simulink library "powerlib_models"  (Simulink 6.0)
settings: Solver=ode45  SolverMode=SingleTasking  StartTime=0.0  StopTime=10.0  RelTol=1e-3
values from neighbouring files (symbols this model uses):
  Ts = get(handles.edit1,'string')    [powergui.m]
undefined symbols (not defined in the file or in its folder): A, a0, a1, a2, a3, a4, a5, Ac, Amplitude, Amplitudes, B, BaseCurrent, BaseFlux, Bc, C, Capacitance, Cc, Columns, ConnectionType, Cs, ctrl, current, Current, damp, Dc, Dd, DiscIntNeverNeededParam, dref, dwo, exc, excAxis, F, Flux, fnom, Frequency, FreqVps, Gain1, gate, GH, GHd, GI, GId, GL, GLd, H, HarmonicGeneration, HT, hyd, I1_init, ib, ib2, Id1o, Inductance, InitialFlux, InitialSlope, io, Iq1o, isfinite, j, J ... (+138)
libraries: powerlib_models x32, powerlib_extras x4
(part 4 of 11)

== system powerlib_models/Discrete/PSS ==
  note: Power System Stabilizer (PSS)
      | (Discrete generic model)
  In : Inport  Port=1  LatchInput=off
  Lead-Lag #1 : Subsystem  AncestorBlock=|  mask(Discrete Lead-Lag Controller){T1=T1n, T2=T1d, V_Init=0, Ts=Ts}
      | powerlib_extras/Discrete 
      | Control Blocks/Discrete
      | Lead-Lag
      mask prompts: T1 "Time constant T1 (s):"; T2 "Time constant T2 (s):"; V_Init "Initial input and output:"; Ts "Sample time (s):"
      mask help:
      | This block implements a discrete lead-lag controller:
      |
      |          1+T1s
      | H(s)= ------
      |          1+T2s
      |
      | States are initialized according to initial input anf output value so that simulation starts in steady state.
      mask init: same as powerlib_models/Discrete/Excitation_System/Lead Lag Compensator tc.s+1 / tb.s+1
      mask Display: disp('1+T1s\n---\n1+T2s')
  Lead-Lag #2 : Subsystem  AncestorBlock=|  mask(Discrete Lead-Lag Controller){T1=T2n, T2=T2d, V_Init=0, Ts=Ts}
      | powerlib_extras/Discrete 
      | Control Blocks/Discrete
      | Lead-Lag
      mask prompts: T1 "Time constant T1 (s):"; T2 "Time constant T2 (s):"; V_Init "Initial input and output:"; Ts "Sample time (s):"
      mask help:
      | This block implements a discrete lead-lag controller:
      |
      |          1+T1s
      | H(s)= ------
      |          1+T2s
      |
      | States are initialized according to initial input anf output value so that simulation starts in steady state.
      mask init: same as powerlib_models/Discrete/Excitation_System/Lead Lag Compensator tc.s+1 / tb.s+1
      mask Display: disp('1+T1s\n---\n1+T2s')
  "Limiter " : Saturate  UpperLimit=VSlimits(2)  LowerLimit=VSlimits(1)
  Overall Gain : Gain  Gain=K  SaturateOnIntegerOverflow=on
  "Sensor " : Subsystem  AncestorBlock=|  mask(Discrete 1st-Order Filter){FilterType=Lowpass, Tc=Tsensor, Ts=Ts, Initialize=on, Vac_Init=[0 0 60], Vdc_Init=Vinit, PlotResponse=off, param1=[1 500 0.1]}
      | powerlib_extras/Discrete 
      | Control Blocks/Discrete
      | 1st-Order
      | Discrete Filter
      mask prompts: FilterType "Filter Type:"; Tc "Time constant (s):"; Ts "Sample time:"; Initialize "Initialize filter states"; Vac_Init "AC initial input: [ Mag  Phase(degrees)  Freq(Hz) ]"; Vdc_Init "DC Initial input:"; PlotResponse "Plot filter response"; param1 "Frequency range(Hz) : [Start  End  Inc.]"
      mask init:
      | switch FilterType
      | case 1, % Lowpass
      |        X=[0 1 2 3 4];
      |        Y=[-2 -2 -3 -4 -4];
      |        numc=1;
      |        denc=[Tc 1];
      |  case 2,   % Highpass
      |        X=[0 1 2 3 4];
      |        Y=[-4 -4 -3 -2 -2];
      |         numc=[1 0];
      |         denc=[1 1/Tc];
      | end
      | %
      | [Ac,Bc,Cc,Dc]=tf2ss(numc,denc);
      | %
      | %  Conversion to discrete transfer function
      | nstates = size(Ac,1);
      | invexp = inv(eye(nstates) - (Ts/2)*Ac);
      | Ad = invexp*(eye(nstates) + (Ts/2)*Ac);
      | Bd = invexp*Bc;
      | Cd = Cc*invexp*Ts;
      | Dd = Cc*invexp*Bc*(Ts/2) + Dc;
      | %
      | if Initialize==1  % Compute initial conditions on states
      | u1=Vac_Init(1)*exp(j*Vac_Init(2)*pi/180);
      | u2=Vdc_Init*exp(j*90*pi/180);
      | u=u1+u2;
      | u0=imag(u); % input at  t=0;
      | I=eye(size(Ac));
      | sI1=I*j*(2*pi*Vac_Init(3));
      | sI2=I*j*0;
      | x=inv(sI1-Ac)*Bc*u1 + inv(sI2-Ac)*Bc*u2;
      | x0c=imag(x);
      | x0d=(I-Ac*Ts/2)*x0c/Ts - Bc/2*u0;
      | else
      | x0d=0;
      | end
      | 
      | %
      | if PlotResponse==1 % Plot frequency and step response
      | figure(1)
      | sys=ss(Ad,Bd,Cd,Dd,Ts);
      | f=param1(1):param1(3):param1(2);
      | w=2*pi*f;
      | [mag phase]=bode(sys,w);
      | subplot(2,1,1)
      | plot(f,squeeze(mag))
      | title('Magnitude')
      | grid
      | subplot(2,1,2)
      | plot(f,squeeze(phase))
      | title('Phase (degrees)')
      | xlabel('Hz')
      | grid
      | figure(2)
      | step(sys)
      | end
      mask StyleString: popup(Lowpass|Highpass),edit,edit,checkbox,edit,edit,checkbox,edit
      mask CallbackString: |||p4=get_param(gcb,'Initialize');if strcmp(p4,'on');visible={'on','on','on','on','on','on','on',get_param(gcb,'PlotResponse')};else;visible={'on','on','on','on','off','off','on',get_param(gcb,'PlotResponse')};end;set_param(gcb,'MaskVisibilities',visible)|||p7=get_param(gcb,'PlotResponse');if strcmp(p7,'on');visible={'on','on','on','on',get_param(gcb,'Initialize'),get_param(gcb,'Initialize'),'on','on'};else;visible={'on','on','on','on',get_param(gcb,'Initialize'),get_param(gcb,'Initialize'),'on','off'};end;set_param(gcb,'MaskVisibilities',visible)|
      mask Display: plot(X,Y);
  "Wash-out " : Subsystem  AncestorBlock=|  mask(Discrete 1st-Order Filter){FilterType=Highpass, Tc=Twashout, Ts=Ts, Initialize=on, Vac_Init=[0 0 60], Vdc_Init=K*Vinit, PlotResponse=off, param1=[1 500 0.1]}
      | powerlib_extras/Discrete 
      | Control Blocks/Discrete
      | 1st-Order
      | Discrete Filter
      mask prompts: FilterType "Filter Type:"; Tc "Time constant (s):"; Ts "Sample time:"; Initialize "Initialize filter states"; Vac_Init "AC initial input: [ Mag  Phase(degrees)  Freq(Hz) ]"; Vdc_Init "DC Initial input:"; PlotResponse "Plot filter response"; param1 "Frequency range(Hz) : [Start  End  Inc.]"
      mask init: same as powerlib_models/Discrete/PSS/Sensor 
      mask StyleString: popup(Lowpass|Highpass),edit,edit,checkbox,edit,edit,checkbox,edit
      mask CallbackString: |||p4=get_param(gcb,'Initialize');if strcmp(p4,'on');visible={'on','on','on','on','on','on','on',get_param(gcb,'PlotResponse')};else;visible={'on','on','on','on','off','off','on',get_param(gcb,'PlotResponse')};end;set_param(gcb,'MaskVisibilities',visible)|||p7=get_param(gcb,'PlotResponse');if strcmp(p7,'on');visible={'on','on','on','on',get_param(gcb,'Initialize'),get_param(gcb,'Initialize'),'on','on'};else;visible={'on','on','on','on',get_param(gcb,'Initialize'),get_param(gcb,'Initialize'),'on','off'};end;set_param(gcb,'MaskVisibilities',visible)|
      mask Display: plot(X,Y);
  VS : Outport  InitialOutput=0
  wires:
  Lead-Lag #1/1(Out1) -> Lead-Lag #2/1(In1)
  In/1 -> "Sensor "/1(In)
  "Sensor "/1(Out) -> Overall Gain/1
  Overall Gain/1 -> "Wash-out "/1(In)
  "Wash-out "/1(Out) -> Lead-Lag #1/1(In1)
  Lead-Lag #2/1(Out1) -> "Limiter "/1
  "Limiter "/1 -> VS/1

== system powerlib_models/Discrete/SM_mechanics ==
  note: This subsystem models the mechanical part of the machine.
  "Te " : Inport  Port=1  PortDimensions=1  LatchInput=off
  Pm : Inport  Port=2  LatchInput=off
  1_(2H) : Gain  Gain=1/(2*H)  SaturateOnIntegerOverflow=on
  1_Pb : Gain  Gain=1/Pb  SaturateOnIntegerOverflow=on
  Clock : Clock
      settings: Decimation=10
  Discrete-Time Integrator : DiscreteIntegrator  InitialCondition=dwo  SampleTime=Ts  ICPrevOutput=DiscIntNeverNeededParam  ICPrevScaledInput=DiscIntNeverNeededParam
  Discrete-Time Integrator1 : DiscreteIntegrator  InitialCondition=tho  SampleTime=Ts  ICPrevOutput=DiscIntNeverNeededParam  ICPrevScaledInput=DiscIntNeverNeededParam
  Discrete-Time Integrator2 : DiscreteIntegrator  InitialCondition=tho  SampleTime=Ts  ICPrevOutput=DiscIntNeverNeededParam  ICPrevScaledInput=DiscIntNeverNeededParam
  F1 : Gain  Orientation=left  Gain=F  SaturateOnIntegerOverflow=on
  Fcn : Fcn  Expr=rem(u,2*pi)
  Mux1 : Mux  Inputs=2
  Mux2 : Mux  Inputs=6
  Product : Product  SaturateOnIntegerOverflow=on  InputSameDT=on
  Sum : Sum  SaturateOnIntegerOverflow=on  InputSameDT=on
  Sum2 : Sum  Inputs=+--  SaturateOnIntegerOverflow=on  InputSameDT=on
  Sum3 : Sum  SaturateOnIntegerOverflow=on  InputSameDT=on
  div : Fcn  Expr=u[2]/u[1]
      mask Display: disp('/')
  nom. speed : Constant
  theta : Gain  Gain=180/pi  SaturateOnIntegerOverflow=on
  units : Gain  Gain=Nb  SaturateOnIntegerOverflow=on
  units1 : Gain  Gain=Pb  SaturateOnIntegerOverflow=on
  units2 : Gain  Gain=Pb/Nb  SaturateOnIntegerOverflow=on
  web1 : Gain  Gain=web_psb  SaturateOnIntegerOverflow=on
  web2 : Gain  Gain=web_psb  SaturateOnIntegerOverflow=on
  web3 : Gain  Gain=web_psb  SaturateOnIntegerOverflow=on
  m : Outport  InitialOutput=0
  theta_e : Outport  Port=2  InitialOutput=0
  we : Outport  Port=3  InitialOutput=0
  wires:
  Discrete-Time Integrator1/1 -> Mux2/1, Sum3/1  "d_theta (rad)"
  web2/1 -> Sum3/2
  Clock/1 -> web2/1
  web1/1 -> Discrete-Time Integrator1/1
  Discrete-Time Integrator/1 -> web1/1, Mux2/4, Sum/2  "dw"
  Product/1 -> units1/1  "Pe"
  nom. speed/1 -> Sum/1
  1_(2H)/1 -> Discrete-Time Integrator/1
  div/1 -> Sum2/1
  "Te "/1 -> Sum2/2, Product/2, units2/1  "Te"
  Mux1/1 -> div/1
  Pm/1 -> 1_Pb/1
  1_Pb/1 -> Mux1/2
  F1/1 -> Sum2/3
  Sum2/1 -> 1_(2H)/1
  Sum/1 -> F1/1, Product/1, web3/1, units/1, we/1, Mux1/1  "n"
  Mux2/1 -> m/1
  Sum3/1 -> theta_e/1
  Fcn/1 -> theta/1
  Discrete-Time Integrator2/1 -> Fcn/1
  web3/1 -> Discrete-Time Integrator2/1
  theta/1 -> Mux2/5  "theta"
  units/1 -> Mux2/2
  units1/1 -> Mux2/3
  units2/1 -> Mux2/6

== system powerlib_models/Discrete/SSM_mechanics ==
  Pm : Inport  Port=1  LatchInput=off
  Pe : Inport  Port=2  LatchInput=off
  1_(2*H) : Gain  Gain=1/(2*H)  SaturateOnIntegerOverflow=on
  1_Pb : Gain  Gain=1/Pb  SaturateOnIntegerOverflow=on
  Discrete-Time Integrator : DiscreteIntegrator  IntegratorMethod=Integration: Trapezoidal  InitialCondition=dwo  SampleTime=Ts  ICPrevOutput=DiscIntNeverNeededParam  ICPrevScaledInput=DiscIntNeverNeededParam
  Discrete-Time Integrator1 : DiscreteIntegrator  IntegratorMethod=Integration: Trapezoidal  InitialCondition=tho  SampleTime=Ts  ICPrevOutput=DiscIntNeverNeededParam  ICPrevScaledInput=DiscIntNeverNeededParam
  Gain : Gain  Orientation=left  Gain=Kd  SaturateOnIntegerOverflow=on
  Mux1 : Mux  Inputs=2
  Predict : Subsystem
  Sum : Sum  SaturateOnIntegerOverflow=on  InputSameDT=on
  Sum1 : Sum  Inputs=+-  SaturateOnIntegerOverflow=on  InputSameDT=on
  Sum2 : Sum  Inputs=-+  SaturateOnIntegerOverflow=on  InputSameDT=on
  Unit Delay2 : UnitDelay  X0=dwo  SampleTime=Ts
  div : Fcn  Expr=u[2]/u[1]
      mask Display: disp('division')
  nom. speed : Constant
  web_psb : Gain  Gain=web_psb  SaturateOnIntegerOverflow=on
  theta_e : Outport  InitialOutput=0
  wm : Outport  Port=2  InitialOutput=0
  wires:
  Predict/1(O) -> Sum/2, Gain/1
  Unit Delay2/1 -> Predict/1(I)
  Pm/1 -> 1_Pb/1
  1_Pb/1 -> Sum2/2
  web_psb/1 -> Discrete-Time Integrator1/1
  Discrete-Time Integrator1/1 -> theta_e/1
  Mux1/1 -> div/1
  Pe/1 -> Sum2/1
  Sum2/1 -> Mux1/2
  Sum/1 -> Mux1/1, wm/1, web_psb/1
  1_(2*H)/1 -> Discrete-Time Integrator/1
  div/1 -> Sum1/1
  Gain/1 -> Sum1/2
  Sum1/1 -> 1_(2*H)/1
  Discrete-Time Integrator/1 -> Unit Delay2/1
  nom. speed/1 -> Sum/1

== system powerlib_models/Discrete/Three-Level Bridge ==
  v : Inport  Port=1  PortDimensions=nb_arm*3  LatchInput=off
  g : Inport  Port=2  PortDimensions=nb_arm*4  LatchInput=off
  2-level GTO-IGBT Bridge  Logic (modified) : Subsystem  AncestorBlock=powerlib_models/Discrete/GTO-IGBT Bridge  mask(GTO & IGBT Bridge Logic(modified)){nb_arm=nb_arm, Tf=0, Tt=0, Cs=Cs, VFs=Par_Vf, Rsw=Ron, Ts=Ts}
      mask prompts: nb_arm "Number of bridge arms (1,2 or 3)"; Tf "Curent 10% fall time Tf (s) :"; Tt "Current tail time Tt (s) :"; Cs "Snubber Capacitance Cs (F):"; VFs "Forward Voltages [ Vf  Vfd ]"; Rsw "Device resistance"; Ts "Time step Ts (s) :"
      mask help:
      | Generates the switch status ( 0 or 1) and the tail currents for a forced-commutated two- level bridge using GTO/Diode or IGBT/Diode pairs.
      | Specify  3 arms (6 switches) for 3 phase bridge, 2 arms for 4 switches, or 1 arm.
      | To turn-off the tail current, specify Tf=0 and Tt=0.
      mask init: same as powerlib_models/Continuous/Three-Level Bridge/2-level GTO-IGBT Bridge  Logic (modified)
  Input : Subsystem
  Mux : Mux  Inputs=[nb_arm*2 nb_arm]
  Mux1 : Mux  Inputs=[nb_arm*2 nb_arm]
  Select_Status : Selector  Elements=StatusElements  InputPortWidth=3*nb_arm
  Select_Status1 : Selector  Elements=StatusElements  InputPortWidth=3*nb_arm
  SubSystem : Subsystem
      mask Display: disp('?')
  Sw3 (clamping diode) Logic : Subsystem  mask{nb_arm=nb_arm, VFs=Par_Vf, Ts=Ts}
      mask prompts: nb_arm "Number of bridge arm:"; VFs "Forward Voltages [ Vf  Vfd ]"; Ts "Sample time:"
      mask init: same as powerlib_models/Continuous/Three-Level Bridge/Sw3 (clamping diode) Logic
  x : Outport
  Status : Outport  Port=2
  Vf : Outport  Port=3
  wires:
  Select_Status1/1 -> Vf/1
  Select_Status/1 -> Status/1, x/1
  2-level GTO-IGBT Bridge  Logic (modified)/3(Block3) -> Sw3 (clamping diode) Logic/3(Block3)
  Sw3 (clamping diode) Logic/4(Block12) -> 2-level GTO-IGBT Bridge  Logic (modified)/3(Block12)
  Sw3 (clamping diode) Logic/3(g12) -> 2-level GTO-IGBT Bridge  Logic (modified)/2(g)
  Sw3 (clamping diode) Logic/2(Vf) -> Mux1/2
  Sw3 (clamping diode) Logic/1(Status) -> Mux/2
  2-level GTO-IGBT Bridge  Logic (modified)/2(Vf) -> Mux1/1
  Mux/1 -> Select_Status/1
  Mux1/1 -> Select_Status1/1
  2-level GTO-IGBT Bridge  Logic (modified)/1(status) -> Mux/1
  v/1 -> Sw3 (clamping diode) Logic/1(V_Sw123), 2-level GTO-IGBT Bridge  Logic (modified)/1(v)
  Sw3 (clamping diode) Logic/5(Trig12) -> 2-level GTO-IGBT Bridge  Logic (modified)/4(Trig12)
  g/1 -> Input/1(In)
  Input/1(Out) -> Sw3 (clamping diode) Logic/2(Pulses)
  2-level GTO-IGBT Bridge  Logic (modified)/4(status_GTO) -> Sw3 (clamping diode) Logic/4(Status_GTO)

== system powerlib_models/Discrete/Xfohyst1Ph ==
  Goto2 : Terminator
  transformer : powerlib_models/Discrete/hysteresis_transformer  SaturationFlux=SaturationFlux  SaturationCurrent=SaturationCurrent  InitialFlux=InitialFlux  FluxBase=BaseFlux  CurrentBase=BaseCurrent  Tolerances=Tolerances  HT=HT  UpperFlux=UpperFlux  LowerFlux=LowerFlux  Current=current  InitialSlope=InitialSlope  TransfoNumber=TransfoNumber  Ts=Ts  sfun_InitialFlux=sfun_InitialFlux
  tag scope: LibraryTag=global
  wires:
  transformer/2 -> Goto2/1
  [LibraryTag] -> transformer/1
  transformer/1 -> [LibraryTag]

== system powerlib_models/Discrete/Xfohyst1PhF ==
  transformer : powerlib_models/Discrete/hysteresis_transformer  SaturationFlux=SaturationFlux  SaturationCurrent=SaturationCurrent  InitialFlux=InitialFlux  FluxBase=BaseFlux  CurrentBase=BaseCurrent  Tolerances=Tolerances  HT=HT  UpperFlux=UpperFlux  LowerFlux=LowerFlux  Current=current  InitialSlope=InitialSlope  TransfoNumber=TransfoNumber  Ts=Ts  sfun_InitialFlux=sfun_InitialFlux
  tag scope: LibraryTag=global
  wires:
  transformer/2 -> [LibraryTag]
  transformer/1 -> [LibraryTag]
  [LibraryTag] -> transformer/1

== system powerlib_models/Discrete/Xfohyst3Ph ==
  Goto2 : Terminator
  Goto4 : Terminator
  Goto6 : Terminator
  transformer1 : powerlib_models/Discrete/hysteresis_transformer  SaturationFlux=SaturationFlux  SaturationCurrent=SaturationCurrent  InitialFlux=InitialFlux1  FluxBase=BaseFlux  CurrentBase=BaseCurrent  Tolerances=Tolerances  HT=HT  UpperFlux=UpperFlux  LowerFlux=LowerFlux  Current=current  InitialSlope=InitialSlope  TransfoNumber=TransfoNumber1  Ts=Ts  sfun_InitialFlux=sfun_InitialFlux1
  transformer2 : powerlib_models/Discrete/hysteresis_transformer  SaturationFlux=SaturationFlux  SaturationCurrent=SaturationCurrent  InitialFlux=InitialFlux2  FluxBase=BaseFlux  CurrentBase=BaseCurrent  Tolerances=Tolerances  HT=HT  UpperFlux=UpperFlux  LowerFlux=LowerFlux  Current=current  InitialSlope=InitialSlope  TransfoNumber=TransfoNumber2  Ts=Ts  sfun_InitialFlux=sfun_InitialFlux2
  transformer3 : powerlib_models/Discrete/hysteresis_transformer  SaturationFlux=SaturationFlux  SaturationCurrent=SaturationCurrent  InitialFlux=InitialFlux3  FluxBase=BaseFlux  CurrentBase=BaseCurrent  Tolerances=Tolerances  HT=HT  UpperFlux=UpperFlux  LowerFlux=LowerFlux  Current=current  InitialSlope=InitialSlope  TransfoNumber=TransfoNumber3  Ts=Ts  sfun_InitialFlux=sfun_InitialFlux3
  tag scope: LibraryTag=global
  wires:
  transformer3/1 -> [LibraryTag]
  transformer2/1 -> [LibraryTag]
  transformer1/1 -> [LibraryTag]
  [LibraryTag] -> transformer3/1
  [LibraryTag] -> transformer2/1
  [LibraryTag] -> transformer1/1
  transformer1/2 -> Goto2/1
  transformer2/2 -> Goto4/1
  transformer3/2 -> Goto6/1

== system powerlib_models/Discrete/Xfohyst3PhF ==
  transformer1 : powerlib_models/Discrete/hysteresis_transformer  SaturationFlux=SaturationFlux  SaturationCurrent=SaturationCurrent  InitialFlux=InitialFlux1  FluxBase=BaseFlux  CurrentBase=BaseCurrent  Tolerances=Tolerances  HT=HT  UpperFlux=UpperFlux  LowerFlux=LowerFlux  Current=current  InitialSlope=InitialSlope  TransfoNumber=TransfoNumber1  Ts=Ts  sfun_InitialFlux=sfun_InitialFlux1
  transformer2 : powerlib_models/Discrete/hysteresis_transformer  SaturationFlux=SaturationFlux  SaturationCurrent=SaturationCurrent  InitialFlux=InitialFlux2  FluxBase=BaseFlux  CurrentBase=BaseCurrent  Tolerances=Tolerances  HT=HT  UpperFlux=UpperFlux  LowerFlux=LowerFlux  Current=current  InitialSlope=InitialSlope  TransfoNumber=TransfoNumber2  Ts=Ts  sfun_InitialFlux=sfun_InitialFlux2
  transformer3 : powerlib_models/Discrete/hysteresis_transformer  SaturationFlux=SaturationFlux  SaturationCurrent=SaturationCurrent  InitialFlux=InitialFlux3  FluxBase=BaseFlux  CurrentBase=BaseCurrent  Tolerances=Tolerances  HT=HT  UpperFlux=UpperFlux  LowerFlux=LowerFlux  Current=current  InitialSlope=InitialSlope  TransfoNumber=TransfoNumber3  Ts=Ts  sfun_InitialFlux=sfun_InitialFlux3
  tag scope: LibraryTag=global
  wires:
  [LibraryTag] -> transformer1/1
  [LibraryTag] -> transformer2/1
  [LibraryTag] -> transformer3/1
  transformer1/1 -> [LibraryTag]
  transformer1/2 -> [LibraryTag]
  transformer2/1 -> [LibraryTag]
  transformer2/2 -> [LibraryTag]
  transformer3/1 -> [LibraryTag]
  transformer3/2 -> [LibraryTag]

== system powerlib_models/Discrete/Xfosat1Ph ==
  Goto2 : Terminator
  transformer : powerlib_models/Discrete/saturable_transformer  SaturationFlux=SaturationFlux  SaturationCurrent=SaturationCurrent  InitialFlux=InitialFlux  Ts=Ts
  tag scope: LibraryTag=global
  wires:
  transformer/1 -> [LibraryTag]
  [LibraryTag] -> transformer/1
  transformer/2 -> Goto2/1

== system powerlib_models/Discrete/Xfosat1PhF ==
  transformer : powerlib_models/Discrete/saturable_transformer  SaturationFlux=SaturationFlux  SaturationCurrent=SaturationCurrent  InitialFlux=InitialFlux  Ts=Ts
  tag scope: LibraryTag=global, tp282148=global
  wires:
  [LibraryTag] -> transformer/1
  transformer/1 -> [LibraryTag]
  transformer/2 -> [tp282148]

== system powerlib_models/Discrete/Xfosat3Ph ==
  Goto2 : Terminator
  Goto4 : Terminator
  Goto6 : Terminator
  transformer1 : powerlib_models/Discrete/saturable_transformer  SaturationFlux=SaturationFlux  SaturationCurrent=SaturationCurrent  InitialFlux=InitialFlux1  Ts=Ts
  transformer2 : powerlib_models/Discrete/saturable_transformer  SaturationFlux=SaturationFlux  SaturationCurrent=SaturationCurrent  InitialFlux=InitialFlux2  Ts=Ts
  transformer3 : powerlib_models/Discrete/saturable_transformer  SaturationFlux=SaturationFlux  SaturationCurrent=SaturationCurrent  InitialFlux=InitialFlux3  Ts=Ts
  tag scope: LibraryTag=global
  wires:
  transformer3/2 -> Goto6/1
  transformer2/2 -> Goto4/1
  transformer1/2 -> Goto2/1
  [LibraryTag] -> transformer1/1
  [LibraryTag] -> transformer2/1
  [LibraryTag] -> transformer3/1
  transformer1/1 -> [LibraryTag]
  transformer2/1 -> [LibraryTag]
  transformer3/1 -> [LibraryTag]

== system powerlib_models/Discrete/Xfosat3PhF ==
  transformer1 : powerlib_models/Discrete/saturable_transformer  SaturationFlux=SaturationFlux  SaturationCurrent=SaturationCurrent  InitialFlux=InitialFlux1  Ts=Ts
  transformer2 : powerlib_models/Discrete/saturable_transformer  SaturationFlux=SaturationFlux  SaturationCurrent=SaturationCurrent  InitialFlux=InitialFlux2  Ts=Ts
  transformer3 : powerlib_models/Discrete/saturable_transformer  SaturationFlux=SaturationFlux  SaturationCurrent=SaturationCurrent  InitialFlux=InitialFlux3  Ts=Ts
  tag scope: LibraryTag=global
  wires:
  transformer3/2 -> [LibraryTag]
  transformer3/1 -> [LibraryTag]
  transformer2/2 -> [LibraryTag]
  transformer2/1 -> [LibraryTag]
  transformer1/2 -> [LibraryTag]
  transformer1/1 -> [LibraryTag]
  [LibraryTag] -> transformer3/1
  [LibraryTag] -> transformer2/1
  [LibraryTag] -> transformer1/1

== system powerlib_models/Discrete/asynchronous_machine ==
  v : Inport  Port=1  LatchInput=off
  thr,wr : Inport  Port=2  LatchInput=off
  Gain : Gain  Gain=[ib2*ones(5,1);phib2;phib2;Vb2;Vb2;ib2*ones(5,1);phib2;phib2;Vb2;Vb2]  SaturateOnIntegerOverflow=on
  Mutual fluxes : Subsystem  Orientation=left
  Mux3 : Mux  Inputs=[3,2,2,2,3,2,2,2]
  Product1 : Product  Inputs=1  SaturateOnIntegerOverflow=on  InputSameDT=on
  Product2 : Product  Inputs=1  SaturateOnIntegerOverflow=on  InputSameDT=on
  Rotor : Subsystem
      mask Display: disp('Rotor')
  Selector : Selector  Elements=[1 4]  InputPortWidth=4
  Selector1 : Selector  Elements=[2 3]  InputPortWidth=4
  Stator : Subsystem
      mask Display: disp('Stator')
  Sum1 : Sum  Inputs=|-+  SaturateOnIntegerOverflow=on  InputSameDT=on
  abc2qd : Subsystem
      mask Display: disp('abc2qd')
  dq2abc : Subsystem
  sin,cos : Subsystem
  i : Outport
  m : Outport  Port=2
  Te : Outport  Port=3
  wires:
  sin,cos/2(w-wr) -> Rotor/2(w-wr)
  Mutual fluxes/1(phimq,phimd) -> Rotor/3(phimq,phimd), Stator/1(phimq,phimd)
  sin,cos/1(sin,cos) -> abc2qd/2(sin,cos), dq2abc/1(sin,cos)
  sin,cos/3(w) -> Stator/3(w)
  abc2qd/2(vqs,vds) -> Stator/2(vqs,vds), Mux3/8
  abc2qd/1(vqr,vdr) -> Rotor/1(vqr,vdr), Mux3/4
  dq2abc/1(irab,isab) -> i/1
  Rotor/2(phiqr,phidr) -> Mutual fluxes/1(phiqr,phidr), Mux3/3
  Rotor/1(iqr,idr) -> Mux3/2, dq2abc/2(iqr,idr)
  v/1 -> abc2qd/1(v)
  Stator/1(phiqs,phids) -> Mutual fluxes/2(phiqs,phids), Mux3/7
  Stator/2(iqs,ids) -> dq2abc/3(iqs,ids), Mux3/6
  Mux3/1 -> Gain/1
  Gain/1 -> m/1
  dq2abc/3(isabc) -> Mux3/5
  dq2abc/2(irabc) -> Mux3/1
  Stator/3(phis,is) -> Selector/1, Selector1/1
  thr,wr/1 -> sin,cos/1(thr,wr)
  Selector/1 -> Product1/1
  Selector1/1 -> Product2/1
  Product2/1 -> Sum1/2
  Product1/1 -> Sum1/1
  Sum1/1 -> Te/1

== system powerlib_models/Discrete/breaker ==
  note: Zero crossing detection
  note: Current Prediction
  v : Inport  Port=1  LatchInput=off
  g : Inport  Port=2  LatchInput=off
  0 1 : Constant  Value=0
  >1.5 : Relay  OnSwitchValue=1.5  OffSwitchValue=0
  Constant : Constant  Value=zeros(Nsw,1)
  Data Type  Conversion : DataTypeConversion  OutDataTypeMode=double  SaturateOnIntegerOverflow=on  RndMeth=Zero
  Data Type  Conversion1 : DataTypeConversion  OutDataTypeMode=boolean  SaturateOnIntegerOverflow=on  RndMeth=Zero
  Data Type  Conversion2 : DataTypeConversion  OutDataTypeMode=double  SaturateOnIntegerOverflow=on  RndMeth=Zero
  Data Type  Conversion3 : DataTypeConversion  OutDataTypeMode=boolean  SaturateOnIntegerOverflow=on  RndMeth=Zero
  Data Type  Conversion4 : DataTypeConversion  Orientation=up  OutDataTypeMode=double  SaturateOnIntegerOverflow=on  RndMeth=Zero
  Delay Ts : UnitDelay  SampleTime=Ts
  "Delay Ts " : UnitDelay  SampleTime=Ts
  Delay Ts 1 : UnitDelay  SampleTime=Ts
  Gain : Gain  Gain=2  SaturateOnIntegerOverflow=on
  IC : InitialCondition  Value=istate
  Product : Product  SaturateOnIntegerOverflow=on  InputSameDT=on
  Sum : Sum  Inputs=+-  SaturateOnIntegerOverflow=on  InputSameDT=on
  b5 : RelationalOperator  Operator=>  InputSameDT=on
  or : Logic  Operator=OR
  sum : Sum  SaturateOnIntegerOverflow=on  InputSameDT=on
  i : Outport  InitialOutput=0
  Status : Outport  Port=2  InitialOutput=0
  wires:
  Data Type  Conversion4/1 -> sum/2
  Product/1 -> b5/1
  b5/1 -> Data Type  Conversion2/1
  Data Type  Conversion/1 -> IC/1
  or/1 -> Data Type  Conversion/1
  IC/1 -> Status/1
  Data Type  Conversion1/1 -> or/1
  Delay Ts 1/1 -> Data Type  Conversion1/1
  Data Type  Conversion3/1 -> or/2
  >1.5/1 -> Delay Ts 1/1
  g/1 -> Data Type  Conversion4/1, Data Type  Conversion3/1
  Constant/1 -> i/1
  sum/1 -> >1.5/1
  Data Type  Conversion2/1 -> sum/1
  0 1/1 -> b5/2
  "Delay Ts "/1 -> Product/2
  Sum/1 -> "Delay Ts "/1, Product/1
  v/1 -> Delay Ts/1, Gain/1  "Braeker voltage"
  Delay Ts/1 -> Sum/2
  Gain/1 -> Sum/1

== system powerlib_models/Discrete/detailed_thyristor (logical) ==
  note: Current prediction
  v : Inport  Port=1  LatchInput=off
  g : Inport  Port=2  LatchInput=off
  " Delay Ts1" : UnitDelay  SampleTime=Ts
  " Delay Ts2" : UnitDelay  SampleTime=Ts
  0 {1..4} (4 alike) : Constant  Value=0
  1/Rsw : Gain  Gain=1/Rsw  SaturateOnIntegerOverflow=on
  Constant : Constant  Value=zeros(Nsw,1)
  Data Type  Conversion1 : DataTypeConversion  OutDataTypeMode=double  SaturateOnIntegerOverflow=on  RndMeth=Zero
  Data Type  Conversion{2..5} (4 alike) : DataTypeConversion  OutDataTypeMode=boolean  SaturateOnIntegerOverflow=on  RndMeth=Zero
  Gain : Gain  Gain=2  SaturateOnIntegerOverflow=on
  Mux : Mux  Inputs=2
  Saturation : Saturate  UpperLimit=inf  LowerLimit=0
  Sum : Sum  Inputs=+-  SaturateOnIntegerOverflow=on  InputSameDT=on
  Sum1 : Sum  Inputs=|++  SaturateOnIntegerOverflow=on  InputSameDT=on
  Switch : Switch  Threshold=0.5  InputSameDT=on
  b5 : RelationalOperator  Operator=>  InputSameDT=on
  b6 : RelationalOperator  Operator=>  InputSameDT=on
  b7 : RelationalOperator  Operator===  InputSameDT=on
  or2 : Logic  Operator=OR
  or3 : Logic  Inputs=3
  vf : Constant  Value=Vf
  i : Outport  InitialOutput=0
  Status : Outport  Port=2  InitialOutput=0
  m : Outport  Port=3  InitialOutput=0
  Vf : Outport  Port=4  InitialOutput=0
  wires:
  0 3/1 -> b7/2
  v/1 -> b6/1, Sum1/1, 1/Rsw/1  "Vak"
  0 2/1 -> b6/2
  Gain/1 -> Sum/1
  " Delay Ts1"/1 -> Sum/2
  0 1/1 -> b5/2
  Sum/1 -> b5/1
  or3/1 -> or2/2
  Mux/1 -> m/1  "measurement signals"
  Constant/1 -> i/1
  Sum1/1 -> Mux/2
  vf/1 -> Sum1/2, Vf/1
  or2/1 -> Data Type  Conversion1/1
  Data Type  Conversion1/1 -> " Delay Ts2"/1
  " Delay Ts2"/1 -> Status/1, Switch/2
  g/1 -> Data Type  Conversion2/1
  Data Type  Conversion2/1 -> or3/2
  b7/1 -> Data Type  Conversion3/1
  Data Type  Conversion3/1 -> or3/3
  b6/1 -> Data Type  Conversion4/1
  Data Type  Conversion4/1 -> or3/1
  b5/1 -> Data Type  Conversion5/1
  Data Type  Conversion5/1 -> or2/1
  Switch/1 -> Saturation/1
  Saturation/1 -> Mux/1, b7/1, Gain/1, " Delay Ts1"/1
  1/Rsw/1 -> Switch/1  "Iak"
  0 4/1 -> Switch/3

== system powerlib_models/Discrete/diode (logical) ==
  note: Current Prediction
  v : Inport  Port=1  LatchInput=off
  " Delay Ts" : UnitDelay  SampleTime=Ts
  " Delay Ts1" : UnitDelay  SampleTime=Ts
  0 {1..4} (4 alike) : Constant  Value=0
  1/Rsw : Gain  Gain=1./Rsw  SaturateOnIntegerOverflow=on
  Constant : Constant  Value=zeros(Nsw,1)
  Data Type  Conversion1 : DataTypeConversion  OutDataTypeMode=double  SaturateOnIntegerOverflow=on  RndMeth=Zero
  Gain : Gain  Gain=2  SaturateOnIntegerOverflow=on
  Mux : Mux  Inputs=2
  Saturation : Saturate  UpperLimit=inf  LowerLimit=0
  Sum : Sum  Inputs=+-  SaturateOnIntegerOverflow=on  InputSameDT=on
  Sum1 : Sum  Inputs=|++  SaturateOnIntegerOverflow=on  InputSameDT=on
  Switch : Switch  Threshold=0.5  InputSameDT=on
  b5 : RelationalOperator  Operator=>  InputSameDT=on
  b6 : RelationalOperator  Operator=>  InputSameDT=on
  b7 : RelationalOperator  Operator===  InputSameDT=on
  or2 : Logic  Operator=OR
  or3 : Logic
  vf : Constant  Value=Vf
  i : Outport  InitialOutput=0
  Status : Outport  Port=2  InitialOutput=0
  m : Outport  Port=3  InitialOutput=0
  Vf : Outport  Port=4  InitialOutput=0
  wires:
  Mux/1 -> m/1  "measurement signals"
  b5/1 -> or2/1
  Sum/1 -> b5/1
  0 1/1 -> b5/2
  " Delay Ts"/1 -> Sum/2
  Gain/1 -> Sum/1
  0 2/1 -> b6/2
  v/1 -> b6/1, Sum1/1, 1/Rsw/1  "Vak"
  0 3/1 -> b7/2
  or3/1 -> or2/2
  b6/1 -> or3/1
  b7/1 -> or3/2
  Constant/1 -> i/1
  Sum1/1 -> Mux/2
  vf/1 -> Sum1/2, Vf/1
  or2/1 -> Data Type  Conversion1/1
  Data Type  Conversion1/1 -> " Delay Ts1"/1
  " Delay Ts1"/1 -> Status/1, Switch/2
  1/Rsw/1 -> Switch/1  "Iak"
  Switch/1 -> Saturation/1
  Saturation/1 -> Mux/1, b7/1, Gain/1, " Delay Ts"/1
  0 4/1 -> Switch/3

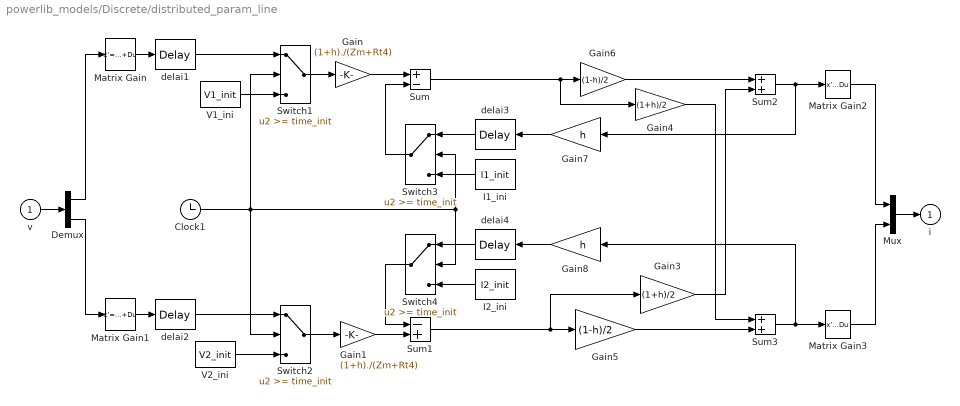
== system powerlib_models/Discrete/distributed_param_line ==
  v : Inport  Port=1  LatchInput=off
  Clock1 : Clock
      settings: Decimation=10
  Demux : Demux  Outputs=[nphase,nphase]
  Gain : Gain  Gain=(1+h)./(Zm+Rt4)  SaturateOnIntegerOverflow=on
  Gain1 : Gain  Gain=(1+h)./(Zm+Rt4)  SaturateOnIntegerOverflow=on
  Gain3 : Gain  Gain=(1+h)/2  SaturateOnIntegerOverflow=on
  Gain4 : Gain  Gain=(1+h)/2  SaturateOnIntegerOverflow=on
  Gain5 : Gain  Gain=(1-h)/2  SaturateOnIntegerOverflow=on
  Gain6 : Gain  Gain=(1-h)/2  SaturateOnIntegerOverflow=on
  Gain7 : Gain  Orientation=left  Gain=h  SaturateOnIntegerOverflow=on
  Gain8 : Gain  Orientation=left  Gain=h  SaturateOnIntegerOverflow=on
  I1_ini : FromWorkspace  Orientation=left  VariableName=I1_init  SampleTime=0
  I2_ini : FromWorkspace  Orientation=left  VariableName=I2_init  SampleTime=0
  Matrix Gain : StateSpace  A=[]  B=[]  C=[]  D=K  mask(Matrix Gain){@1=Ti'}
      mask prompts: @1 "Gain matrix:"
      mask help: Matrix Gain.
      mask init:
      | K = @1;
      mask Help: Multiplies input vector by entered matrix to produce output vector (y=Au).
      mask Display: disp('K')
  Matrix Gain1 : StateSpace  A=[]  B=[]  C=[]  D=K  mask(Matrix Gain){@1=Ti'}
      mask prompts: @1 "Gain matrix:"
      mask help: Matrix Gain.
      mask init:
      | K = @1;
      mask Help: Multiplies input vector by entered matrix to produce output vector (y=Au).
      mask Display: disp('K')
  Matrix Gain2 : StateSpace  A=[]  B=[]  C=[]  D=K  mask(Matrix Gain){@1=Ti}
      mask prompts: @1 "Gain matrix:"
      mask help: Matrix Gain.
      mask init:
      | K = @1;
      mask Help: Multiplies input vector by entered matrix to produce output vector (y=Au).
      mask Display: disp('K')
  Matrix Gain3 : StateSpace  A=[]  B=[]  C=[]  D=K  mask(Matrix Gain){@1=Ti}
      mask prompts: @1 "Gain matrix:"
      mask help: Matrix Gain.
      mask init:
      | K = @1;
      mask Help: Multiplies input vector by entered matrix to produce output vector (y=Au).
      mask Display: disp('K')
  Mux : Mux  Inputs=[nphase,nphase]
  Sum : Sum  Inputs=+-  SaturateOnIntegerOverflow=on  InputSameDT=on
  Sum1 : Sum  Inputs=-+  SaturateOnIntegerOverflow=on  InputSameDT=on
  Sum2 : Sum  SaturateOnIntegerOverflow=on  InputSameDT=on
  Sum3 : Sum  SaturateOnIntegerOverflow=on  InputSameDT=on
  Switch1 : Switch  Threshold=time_init  InputSameDT=on
  Switch2 : Switch  Threshold=time_init  InputSameDT=on
  Switch3 : Switch  Orientation=left  Threshold=time_init  InputSameDT=on
  Switch4 : Switch  Orientation=left  Threshold=time_init  InputSameDT=on
  V1_ini : FromWorkspace  VariableName=V1_init  SampleTime=0
  V2_ini : FromWorkspace  VariableName=V2_init  SampleTime=0
  delai1 : TransportDelay  DelayTime=to
  delai2 : TransportDelay  DelayTime=to
  delai3 : TransportDelay  Orientation=left  DelayTime=to
  delai4 : TransportDelay  Orientation=left  DelayTime=to
  i : Outport  InitialOutput=0
  wires:
  I2_ini/1 -> Switch4/3
  I1_ini/1 -> Switch3/3
  Clock1/1 -> Switch3/2, Switch4/2, Switch1/2, Switch2/2
  delai4/1 -> Switch4/1
  Switch4/1 -> Sum1/1
  Switch3/1 -> Sum/2
  delai3/1 -> Switch3/1
  Sum1/1 -> Gain5/1, Gain3/1
  Sum/1 -> Gain6/1, Gain4/1
  V2_ini/1 -> Switch2/3
  delai2/1 -> Switch2/1
  Switch1/1 -> Gain/1
  Switch2/1 -> Gain1/1
  V1_ini/1 -> Switch1/3
  delai1/1 -> Switch1/1
  Gain8/1 -> delai4/1
  Gain7/1 -> delai3/1
  Mux/1 -> i/1
  v/1 -> Demux/1
  Gain1/1 -> Sum1/2
  Gain/1 -> Sum/1
  Gain5/1 -> Sum3/2
  Gain6/1 -> Sum2/1
  Gain3/1 -> Sum2/2
  Gain4/1 -> Sum3/1
  Matrix Gain/1 -> delai1/1
  Demux/1 -> Matrix Gain/1
  Matrix Gain1/1 -> delai2/1
  Demux/2 -> Matrix Gain1/1
  Matrix Gain3/1 -> Mux/2
  Matrix Gain2/1 -> Mux/1
  Sum3/1 -> Matrix Gain3/1, Gain8/1
  Sum2/1 -> Matrix Gain2/1, Gain7/1

== system powerlib_models/Discrete/hysteresis_transformer ==
  v : Inport  Port=1  LatchInput=off
  Hysteresis ( always in SI ) : Subsystem
  fluxinit : DiscreteIntegrator  IntegratorMethod=Integration: Backward Euler  InitialCondition=InitialFlux  SampleTime=Ts  ICPrevOutput=DiscIntNeverNeededParam  ICPrevScaledInput=DiscIntNeverNeededParam
  i : Outport  InitialOutput=0
  f : Outport  Port=2  InitialOutput=0
  wires:
  v/1 -> fluxinit/1
  fluxinit/1 -> f/1, Hysteresis ( always in SI )/1(In1)  "flux displayed by Multimeter block"
  Hysteresis ( always in SI )/1(Out1) -> i/1

== system powerlib_models/Discrete/ideal_switch ==
  v : Inport  Port=1  LatchInput=off
  g : Inport  Port=2  LatchInput=off
  0 1 : Constant  Value=0
  1/Rsw : Gain  Gain=1./Rsw  SaturateOnIntegerOverflow=on
  Constant : Constant  Value=zeros(Nsw,1)
  Data Type Conversion : DataTypeConversion  OutDataTypeMode=double  SaturateOnIntegerOverflow=on  RndMeth=Zero
  Mux : Mux  Inputs=2
  Switch : Switch  Threshold=0.5  InputSameDT=on
  i : Outport  InitialOutput=0
  Status : Outport  Port=2  InitialOutput=0
  m : Outport  Port=3  InitialOutput=0
  wires:
  v/1 -> 1/Rsw/1, Mux/2  "Vak"
  Mux/1 -> m/1  "measurement signals"
  g/1 -> Switch/2, Data Type Conversion/1
  Constant/1 -> i/1
  Switch/1 -> Mux/1
  1/Rsw/1 -> Switch/1  "Iak"
  0 1/1 -> Switch/3
  Data Type Conversion/1 -> Status/1

== system powerlib_models/Discrete/saturable_transformer ==
  v : Inport  Port=1  LatchInput=off
  Discrete-Time Integrator : DiscreteIntegrator  IntegratorMethod=Integration: Trapezoidal  InitialCondition=InitialFlux  SampleTime=Ts  ICPrevOutput=DiscIntNeverNeededParam  ICPrevScaledInput=DiscIntNeverNeededParam
  Look-Up Table : Lookup  DialogController=Simulink.DDGSource  InputValues=SaturationFlux  OutputValues=SaturationCurrent  SaturateOnIntegerOverflow=on
  i : Outport  InitialOutput=0
  f : Outport  Port=2  InitialOutput=0
  wires:
  v/1 -> Discrete-Time Integrator/1
  Discrete-Time Integrator/1 -> Look-Up Table/1, f/1  "Flux"
  Look-Up Table/1 -> i/1  "Current"

== system powerlib_models/Discrete/simplified_sync_mach ==
  v : Inport  Port=1  LatchInput=off
  e : Inport  Port=2  LatchInput=off
  theta_e : Inport  Port=3  LatchInput=off
  wm : Inport  Port=4  LatchInput=off
  1\p : Gain  Gain=1/p  SaturateOnIntegerOverflow=on
  Selector : Selector  Elements=sel  InputPortWidth=3
  Subsystem : Subsystem
  Vt : Subsystem
  Z : Subsystem
      mask Display: disp('Z')
  gen : Subsystem
      mask Display: disp('gen')
  ib : Gain  Gain=ib  SaturateOnIntegerOverflow=on
  wattmeter : Subsystem  Orientation=left
      mask Display: disp('wattmeter')
  i : Outport  InitialOutput=0
  m : Outport  Port=2  InitialOutput=0
  Pe : Outport  Orientation=left  Port=3  InitialOutput=0
  wires:
  Subsystem/1(*) -> m/1
  Vt/2(Vabc) -> Subsystem/2(v), Z/2(v)
  Vt/1(Vn) -> gen/3(Vn)
  gen/1(e) -> wattmeter/2(v), Z/1(e), Subsystem/3(e)  "e"
  Z/1(i) -> wattmeter/1(i), Subsystem/1(i), ib/1
  wm/1 -> Subsystem/5(wm)
  1\p/1 -> Subsystem/4(theta)
  v/1 -> Vt/1(V)
  theta_e/1 -> gen/1(theta), 1\p/1
  e/1 -> gen/2(E)
  wattmeter/1(Pe) -> Pe/1, Subsystem/6(Pe)
  ib/1 -> Selector/1
  Selector/1 -> i/1

== system powerlib_models/Discrete/surge_arrester ==
  v : Inport  Port=1  LatchInput=off
  Abs : Abs  SaturateOnIntegerOverflow=on
  Product : Product  SaturateOnIntegerOverflow=on  InputSameDT=on
  Sign : Signum  Orientation=down
  Switch1 : Switch  Threshold=ic1  InputSameDT=on
  Switch2 : Switch  Threshold=ic2  InputSameDT=on
  Unit Delay1 : UnitDelay  SampleTime=Ts
  segment1 : Fcn  Expr=p1*(u/uref)^a1
  segment2 : Fcn  Expr=p2*(u/uref)^a2
  segment3 : Fcn  Expr=p3*(u/uref)^a3
  i : Outport  InitialOutput=0
  wires:
  segment3/1 -> Switch2/1
  Switch1/1 -> Switch2/3, Switch2/2
  Switch2/1 -> Product/1
  segment2/1 -> Switch1/1
  segment1/1 -> Switch1/2, Switch1/3
  Abs/1 -> segment3/1, segment2/1, segment1/1
  Sign/1 -> Product/2
  v/1 -> Abs/1, Sign/1
  Product/1 -> Unit Delay1/1
  Unit Delay1/1 -> i/1

== system powerlib_models/Discrete/surge_arrester_directFT ==
  v : Inport  Port=1  LatchInput=off
  Abs : Abs  SaturateOnIntegerOverflow=on
  Product : Product  SaturateOnIntegerOverflow=on  InputSameDT=on
  Sign : Signum  Orientation=down
  Switch1 : Switch  Threshold=ic1  InputSameDT=on
  Switch2 : Switch  Threshold=ic2  InputSameDT=on
  segment1 : Fcn  Expr=p1*(u/uref)^a1
  segment2 : Fcn  Expr=p2*(u/uref)^a2
  segment3 : Fcn  Expr=p3*(u/uref)^a3
  i : Outport  InitialOutput=0
  wires:
  Product/1 -> i/1
  v/1 -> Sign/1, Abs/1
  Sign/1 -> Product/2
  Abs/1 -> segment1/1, segment2/1, segment3/1
  segment1/1 -> Switch1/3, Switch1/2
  segment2/1 -> Switch1/1
  Switch2/1 -> Product/1
  Switch1/1 -> Switch2/2, Switch2/3
  segment3/1 -> Switch2/1

== system powerlib_models/Discrete/synchronous_machine ==
  v : Inport  Port=1  LatchInput=off
  vf : Inport  Port=2  LatchInput=off
  "theta_e " : Inport  Port=3  LatchInput=off
  we : Inport  Port=4  LatchInput=off
  Delta angle : Subsystem
  Mux : Mux  Inputs=[ 1 1 2 ]
  Mux1 : Mux  Inputs=[ 3 8 2 1 1 1]
  PQ : Subsystem
  Te electrical torque : Fcn  Expr=u[1]*u[3]-u[2]*u[4]
  Unit Delay1 : UnitDelay  Orientation=left  X0=phiqo  SampleTime=Ts
  Unit Delay2 : UnitDelay  Orientation=left  X0=phiqo  SampleTime=Ts
  Vfd : Subsystem
  abc2qd : Subsystem
  currents and mutual fluxes : Subsystem
  ia,ib : Selector  Elements=1:2  InputPortWidth=3
  output formatting : Gain  Gain=[ib2*ones(1,5),N2,ib2,ib2,ib2,phib,phib,Vb2,Vb2,1,1,1]
  phid : Subsystem
      mask Display: disp('phid')
  phifd : Subsystem
      mask Display: disp('phifd')
  phikd : Subsystem
      mask Display: disp('phikd')
  phikq1 : Subsystem
      mask Display: disp('phikq1')
  phikq2 : Subsystem
  phiq : Subsystem
  qd2abc : Subsystem
  vkd : Ground
  vkq2 : Ground
  i : Outport  InitialOutput=0
  m : Outport  Port=2  InitialOutput=0
  Te : Outport  Port=3  InitialOutput=0
  wires:
  Vfd/2(Vfd) -> phifd/1(vfd)
  Vfd/1(Vkq1) -> phikq1/2(vkq1)
  phikq2/1(phikq2) -> currents and mutual fluxes/2(phikq2)
  phikq1/1(phikq1) -> currents and mutual fluxes/5(phikq1)
  phifd/1(phifd) -> currents and mutual fluxes/4(phifd)
  phikd/1(phikd) -> currents and mutual fluxes/6(phikd)
  v/1 -> abc2qd/1(v)
  currents and mutual fluxes/4(phimd) -> Unit Delay2/1
  abc2qd/3(vd) -> phid/3(vd), PQ/2(Vd), Delta angle/2(Vd)
  phid/1(phid) -> phiq/3(phid), currents and mutual fluxes/3(phid), Mux/1  "phid"
  output formatting/1 -> m/1
  ia,ib/1 -> i/1
  Mux1/1 -> output formatting/1
  currents and mutual fluxes/3(iq,id) -> PQ/3(Iq), qd2abc/2(iq,id), Mux/3  "iq,id"
  abc2qd/1(cos,sin) -> qd2abc/1(sin,cos)  "sin,cos"
  abc2qd/4(vq,vd) -> Mux1/3  "vq,vd"
  qd2abc/2(is(pu)) -> Mux1/1  "is(3)"
  currents and mutual fluxes/1(phimq) -> Unit Delay1/1
  qd2abc/1(is(A)) -> ia,ib/1  "iabc"
  phiq/1(phiq) -> phid/2(phiq), currents and mutual fluxes/1(phiq), Mux/2
  vkd/1 -> phikd/2(vkd)
  abc2qd/2(vq) -> phiq/1(vq), PQ/1(Vq), Delta angle/1(Vq)
  currents and mutual fluxes/2("iq,id,ifd, ikq1,ikq2,ikd, phimq,phimd") -> Mux1/2  "iq,id,ifd,ikq1,ikq2,ikd,phimq,phimd"
  vf/1 -> Vfd/1(Vf)
  Unit Delay1/1 -> phikq1/1(phimq), phikq2/2(phimq), phiq/4(phimq)
  Delta angle/1(delta) -> Mux1/4
  PQ/1(Peo) -> Mux1/5
  PQ/2(Qeo) -> Mux1/6
  "theta_e "/1 -> abc2qd/2(theta)
  we/1 -> phiq/2(w), phid/1(w)
  vkq2/1 -> phikq2/1(vkq2)
  Unit Delay2/1 -> phid/4(phimd), phifd/2(phimd), phikd/1(phimd)
  Mux/1 -> Te electrical torque/1
  Te electrical torque/1 -> Te/1

== system powerlib_models/Discrete/thyristor (logical) ==
  note: Current prediction
  v : Inport  Port=1  LatchInput=off
  g : Inport  Port=2  LatchInput=off
  " Delay Ts1" : UnitDelay  SampleTime=Ts
  " Delay Ts2" : UnitDelay  SampleTime=Ts
  0 {1..4} (4 alike) : Constant  Value=0
  1/Rsw : Gain  Gain=1./Rsw  SaturateOnIntegerOverflow=on
  Constant : Constant  Value=zeros(Nsw,1)
  Data Type  Conversion1 : DataTypeConversion  OutDataTypeMode=double  SaturateOnIntegerOverflow=on  RndMeth=Zero
  Data Type  Conversion{2..5} (4 alike) : DataTypeConversion  OutDataTypeMode=boolean  SaturateOnIntegerOverflow=on  RndMeth=Zero
  Gain : Gain  Gain=2  SaturateOnIntegerOverflow=on
  Mux : Mux  Inputs=2
  Saturation : Saturate  UpperLimit=inf  LowerLimit=0
  Sum : Sum  Inputs=+-  SaturateOnIntegerOverflow=on  InputSameDT=on
  Sum1 : Sum  Inputs=|++  SaturateOnIntegerOverflow=on  InputSameDT=on
  Switch : Switch  Threshold=0.5  InputSameDT=on
  b5 : RelationalOperator  Operator=>  InputSameDT=on
  b6 : RelationalOperator  Operator=>  InputSameDT=on
  b7 : RelationalOperator  Operator===  InputSameDT=on
  or2 : Logic  Operator=OR
  or3 : Logic  Inputs=3
  vf : Constant  Value=Vf
  i : Outport  InitialOutput=0
  Status : Outport  Port=2  InitialOutput=0
  m : Outport  Port=3  InitialOutput=0
  Vf : Outport  Port=4  InitialOutput=0
  wires:
  Mux/1 -> m/1  "measurement signals"
  or3/1 -> or2/2
  Sum/1 -> b5/1
  0 1/1 -> b5/2
  " Delay Ts1"/1 -> Sum/2
  Gain/1 -> Sum/1
  0 2/1 -> b6/2
  v/1 -> b6/1, Sum1/1, 1/Rsw/1  "Vak"
  0 3/1 -> b7/2
  Constant/1 -> i/1
  Sum1/1 -> Mux/2
  vf/1 -> Sum1/2, Vf/1
  or2/1 -> Data Type  Conversion1/1
  Data Type  Conversion1/1 -> " Delay Ts2"/1
  " Delay Ts2"/1 -> Status/1, Switch/2
  g/1 -> Data Type  Conversion2/1
  Data Type  Conversion2/1 -> or3/2
  b6/1 -> Data Type  Conversion3/1
  Data Type  Conversion3/1 -> or3/1
  b7/1 -> Data Type  Conversion4/1
  Data Type  Conversion4/1 -> or3/3
  b5/1 -> Data Type  Conversion5/1
  Data Type  Conversion5/1 -> or2/1
  1/Rsw/1 -> Switch/1  "Iak"
  0 4/1 -> Switch/3
  Switch/1 -> Saturation/1
  Saturation/1 -> Mux/1, b7/1, " Delay Ts1"/1, Gain/1

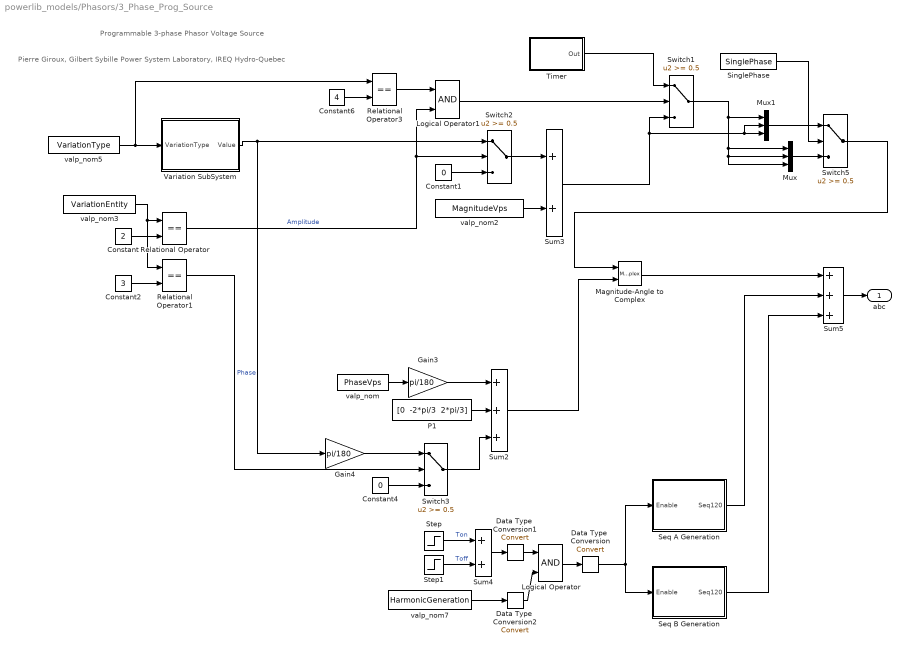
== system powerlib_models/Phasors/3_Phase_Prog_Source ==
  note: Programmable 3-phase Phasor Voltage Source
  note: Pierre Giroux, Gilbert Sybille
      | Power System Laboratory, IREQ
      | Hydro-Quebec
  Constant : Constant  Value=2
  Constant1 : Constant  Value=0
  Constant2 : Constant  Value=3
  Constant4 : Constant  Value=0
  Constant6 : Constant  Value=4
  Data Type  Conversion : DataTypeConversion  OutDataTypeMode=double  SaturateOnIntegerOverflow=on  RndMeth=Zero
  Data Type  Conversion1 : DataTypeConversion  OutDataTypeMode=boolean  SaturateOnIntegerOverflow=on  RndMeth=Zero
  Data Type  Conversion2 : DataTypeConversion  OutDataTypeMode=boolean  SaturateOnIntegerOverflow=on  RndMeth=Zero
  Gain3 : Gain  Gain=pi/180  SaturateOnIntegerOverflow=on
  Gain4 : Gain  Gain=pi/180  SaturateOnIntegerOverflow=on
  Logical Operator : Logic
  Logical Operator1 : Logic
  Magnitude-Angle to Complex : MagnitudeAngleToComplex
  Mux : Mux  Inputs=3
  Mux1 : Mux  Inputs=3
  P1 : Constant  Value="[0  -2*pi/3  2*pi/3]"
  Relational Operator : RelationalOperator  Operator===  InputSameDT=on
  Relational Operator1 : RelationalOperator  Operator===  InputSameDT=on
  Relational Operator3 : RelationalOperator  Operator===  InputSameDT=on
  Seq A Generation : Subsystem  mask(Harmonic generation){Mag_Harmo=Mag_HarmoA *(n_HarmoA==1), Phase_Harmo=Phase_HarmoA, Seq_Harmo=Seq_HarmoA}
  Seq B Generation : Subsystem  mask(Harmonic generation){Mag_Harmo=Mag_HarmoB*(n_HarmoB==1), Phase_Harmo=Phase_HarmoB, Seq_Harmo=Seq_HarmoB}
  SinglePhase : Constant  Value=SinglePhase
  Step : Step  Time=Ton_Harmo  SampleTime=0
  Step1 : Step  Time=Toff_Harmo  After=-1  SampleTime=0
  Sum2 : Sum  Inputs=+++  SaturateOnIntegerOverflow=on  InputSameDT=on
  Sum3 : Sum  SaturateOnIntegerOverflow=on  InputSameDT=on
  Sum4 : Sum  SaturateOnIntegerOverflow=on  InputSameDT=on
  Sum5 : Sum  Inputs=+++  SaturateOnIntegerOverflow=on  InputSameDT=on
  Switch{1..3,5} (4 alike) : Switch  Threshold=0.5  InputSameDT=on
  Timer : Subsystem  mask(Timer){t=TimeValues, e=Amplitudes, Ts=0}
      mask prompts: t "Time (s):"; e "Amplitude:"; Ts "Sample time (s)"
      mask help:
      | Generates a signal changing  at specified times.
      |
      | Value of the signal at time zero must  be specified.
      mask init: same as powerlib_models/Continuous/3_Phase_Prog_Source/Timer
      mask Display: plot( tv(2:end-1), opv(2:end-1) )
  Variation SubSystem : Subsystem  mask(Variation Subsystem){VariationStep=VariationStep, VariationRate=VariationRate, VariationFreq=VariationFrequency, VariationMag=VariationMagnitude, Ton_Variation=Ton_Variation, Toff_Variation=Toff_Variation, Ts=0}
      mask prompts: Ts "Sample time:"
  valp_nom : Constant  Value=PhaseVps  VectorParams1D=off
  valp_nom2 : Constant  Value=MagnitudeVps
  valp_nom3 : Constant  Value=VariationEntity
  valp_nom5 : Constant  Value=VariationType
  valp_nom7 : Constant  Value=HarmonicGeneration
  abc : Outport  InitialOutput=0
  wires:
  Data Type  Conversion/1 -> Seq B Generation/1(Enable), Seq A Generation/1(Enable)
  Seq B Generation/1(Seq120) -> Sum5/3
  Seq A Generation/1(Seq120) -> Sum5/2
  Data Type  Conversion2/1 -> Logical Operator/2
  valp_nom7/1 -> Data Type  Conversion2/1
  Data Type  Conversion1/1 -> Logical Operator/1
  Sum4/1 -> Data Type  Conversion1/1
  Logical Operator/1 -> Data Type  Conversion/1
  P1/1 -> Sum2/2
  Magnitude-Angle to Complex/1 -> Sum5/1
  Gain3/1 -> Sum2/1
  valp_nom/1 -> Gain3/1
  Switch2/1 -> Sum3/1
  Constant1/1 -> Switch2/3
  Sum2/1 -> Magnitude-Angle to Complex/2
  valp_nom2/1 -> Sum3/2
  Relational Operator/1 -> Switch2/2, Logical Operator1/2  "Amplitude"
  valp_nom5/1 -> Variation SubSystem/1(VariationType), Relational Operator3/1
  Switch3/1 -> Sum2/3
  Constant4/1 -> Switch3/3
  Relational Operator1/1 -> Switch3/2  "Phase"
  Variation SubSystem/1(Value) -> Gain4/1, Switch2/1
  Constant/1 -> Relational Operator/2
  valp_nom3/1 -> Relational Operator1/1, Relational Operator/1
  Constant2/1 -> Relational Operator1/2
  Step/1 -> Sum4/1  "Ton"
  Step1/1 -> Sum4/2  "Toff"
  Gain4/1 -> Switch3/1
  Constant6/1 -> Relational Operator3/2
  Sum3/1 -> Switch1/3, Mux1/3, Mux1/2
  Timer/1(Out) -> Switch1/1
  Mux1/1 -> Switch5/1
  SinglePhase/1 -> Switch5/2
  Mux/1 -> Switch5/3
  Switch1/1 -> Mux/1, Mux/2, Mux/3, Mux1/1
  Switch5/1 -> Magnitude-Angle to Complex/1
  Relational Operator3/1 -> Logical Operator1/1
  Logical Operator1/1 -> Switch1/2
  Sum5/1 -> abc/1

== system powerlib_models/Phasors/ASM_mechanics ==
  Tm : Inport  Port=1  LatchInput=off
  Te : Inport  Port=2  LatchInput=off
  1\p : Gain  Gain=1/p  SaturateOnIntegerOverflow=on
  1\p1 : Gain  Gain=[Nb2;Tb2;1]  SaturateOnIntegerOverflow=on
  1_2H : Gain  Gain=1/(2*H)  SaturateOnIntegerOverflow=on
  1_Tb2 : Gain  Gain=1/Tb2  SaturateOnIntegerOverflow=on
  F : Gain  Orientation=left  Gain=F  SaturateOnIntegerOverflow=on
  Integrator : Integrator  InitialCondition=wmo
  Integrator1 : Integrator  InitialCondition=tho
  Mux4 : Mux  Inputs=3
  Sum : Sum  Inputs=-+-  SaturateOnIntegerOverflow=on  InputSameDT=on
  web : Gain  Gain=web_psb  SaturateOnIntegerOverflow=on
  m : Outport
  wr : Outport  Port=2
  wires:
  Te/1 -> Mux4/2, Sum/2
  Integrator1/1 -> 1\p/1
  1\p/1 -> Mux4/3
  web/1 -> Integrator1/1
  1_Tb2/1 -> Sum/1  "Tm"
  F/1 -> Sum/3
  Integrator/1 -> web/1, F/1, Mux4/1, wr/1  "w (pu)"
  1_2H/1 -> Integrator/1
  Sum/1 -> 1_2H/1
  Tm/1 -> 1_Tb2/1
  Mux4/1 -> 1\p1/1
  1\p1/1 -> m/1

== system powerlib_models/Phasors/Dynamic_Load ==
  v : Inport  Port=1  LatchInput=off
  PQ : Inport  Port=2  LatchInput=off
  " filter1" : TransferFcn  Denominator=[1e-3 1]
  Break  Alg. Loop I1 : Subsystem  Orientation=left
  Complex to Real-Imag1 : ComplexToRealImag
  Demux3 : Demux  Outputs=2
  "I1 " : Subsystem
  Mux1 : Mux  Inputs=3
  PQ_ext : Constant  Value=PQext
  Phase currents : Subsystem  Orientation=left
  Power : Subsystem
  Real-Imag to Complex : RealImagToComplex
  Switch1 : Switch  Threshold=0.5  InputSameDT=on
  V> pu : Gain  Gain=1/Vbase  SaturateOnIntegerOverflow=on
  i : Outport  Orientation=left
  m : Outport  Port=2
  wires:
  Phase currents/1(Ia Ib cmplx) -> i/1
  Power/1(P+jQ) -> Switch1/3
  Break  Alg. Loop I1/1(Out) -> Phase currents/1(I1)
  v/1 -> V> pu/1
  "I1 "/1(|V1|) -> " filter1"/1, Power/1(V1)
  V> pu/1 -> "I1 "/1(Vab Vbc cmplx)
  "I1 "/2(I1) -> Break  Alg. Loop I1/1(In)
  " filter1"/1 -> Mux1/1
  Mux1/1 -> m/1
  Complex to Real-Imag1/1 -> Mux1/2
  Complex to Real-Imag1/2 -> Mux1/3
  PQ_ext/1 -> Switch1/2
  Switch1/1 -> "I1 "/2(S=P+jQ), Complex to Real-Imag1/1
  Real-Imag to Complex/1 -> Switch1/1
  Demux3/1 -> Real-Imag to Complex/1
  Demux3/2 -> Real-Imag to Complex/2
  PQ/1 -> Demux3/1

== system powerlib_models/Phasors/Impedance Measurement ==
  v : Inport  Port=1  LatchInput=off
  Constant : Constant  Value=complex(0,0)
  Terminator : Terminator
  i : Outport  InitialOutput=0
  wires:
  Constant/1 -> i/1
  v/1 -> Terminator/1

== system powerlib_models/Phasors/Measurement_MagnitudeAngle ==
  cplx : Inport  Port=1  LatchInput=off
  180/pi : Gain  Gain=180/pi  SaturateOnIntegerOverflow=on
  Complex to Magnitude-Angle : ComplexToMagnitudeAngle
  Mux1 : Mux  Inputs=2
  MA : Outport
  wires:
  Complex to Magnitude-Angle/2 -> 180/pi/1
  180/pi/1 -> Mux1/2
  Complex to Magnitude-Angle/1 -> Mux1/1
  cplx/1 -> Complex to Magnitude-Angle/1
  Mux1/1 -> MA/1

== system powerlib_models/Phasors/Measurement_RealImag ==
  cplx : Inport  Port=1  LatchInput=off
  Complex to Real-Imag : ComplexToRealImag
  Mux2 : Mux  Inputs=2
  ReIm : Outport
  wires:
  Complex to Real-Imag/1 -> Mux2/1
  Complex to Real-Imag/2 -> Mux2/2
  cplx/1 -> Complex to Real-Imag/1
  Mux2/1 -> ReIm/1
